simulink model "FL_simulink"  (R2023b)
settings: Solver=VariableStepAuto  StartTime=0.0  StopTime=30  RelTol=1e-3
values from neighbouring files (symbols this model uses):
  g = 9.81    [ASMC_with_sensor_noise_matlab.m]    (also in ASMC_without_sensor_noise_matlab.m; FL_matlab.m)
  k1 = K(1,1)    [ASMC_with_sensor_noise_matlab.m]    (also in ASMC_without_sensor_noise_matlab.m; FL_matlab.m = K(1))
  k2 = K(2,2)    [ASMC_with_sensor_noise_matlab.m]    (also in ASMC_without_sensor_noise_matlab.m; FL_matlab.m = K(2))
  k3 = K(3,3)    [ASMC_with_sensor_noise_matlab.m]    (also in ASMC_without_sensor_noise_matlab.m; FL_matlab.m = K(3))
  k4 = K(4,4)    [ASMC_with_sensor_noise_matlab.m]    (also in ASMC_without_sensor_noise_matlab.m; FL_matlab.m = K(4))
  k_psi1 = 30    [FL_matlab.m]
  k_psi2 = 50    [FL_matlab.m]
  l = 1    [ASMC_with_sensor_noise_matlab.m]    (also in ASMC_without_sensor_noise_matlab.m; FL_matlab.m)
  phi_0 = pi/6    (= 0.523598775598)    [ASMC_with_sensor_noise_matlab.m]    (also in ASMC_without_sensor_noise_matlab.m; FL_matlab.m)
  psi_0 = pi/6    (= 0.523598775598)    [ASMC_with_sensor_noise_matlab.m]    (also in ASMC_without_sensor_noise_matlab.m; FL_matlab.m)
  psi_d = 0    [ASMC_with_sensor_noise_matlab.m]    (also in ASMC_without_sensor_noise_matlab.m; FL_matlab.m)
  theta_0 = pi/6    (= 0.523598775598)    [ASMC_with_sensor_noise_matlab.m]    (also in ASMC_without_sensor_noise_matlab.m; FL_matlab.m)
  x_0 = 10    [ASMC_with_sensor_noise_matlab.m]    (also in ASMC_without_sensor_noise_matlab.m; FL_matlab.m)
  x_d1 = 20    [ASMC_with_sensor_noise_matlab.m]    (also in ASMC_without_sensor_noise_matlab.m; FL_matlab.m)
  x_d2 = 0    [ASMC_with_sensor_noise_matlab.m]    (also in ASMC_without_sensor_noise_matlab.m; FL_matlab.m)
  y_0 = 10    [ASMC_with_sensor_noise_matlab.m]    (also in ASMC_without_sensor_noise_matlab.m; FL_matlab.m)
  y_d1 = -10    [ASMC_with_sensor_noise_matlab.m]    (also in ASMC_without_sensor_noise_matlab.m; FL_matlab.m)
  y_d2 = 0    [ASMC_with_sensor_noise_matlab.m]    (also in ASMC_without_sensor_noise_matlab.m; FL_matlab.m)
  z_0 = 20    [ASMC_with_sensor_noise_matlab.m]    (also in ASMC_without_sensor_noise_matlab.m; FL_matlab.m)
  z_d1 = 10    [ASMC_with_sensor_noise_matlab.m]    (also in ASMC_without_sensor_noise_matlab.m; FL_matlab.m)
  z_d2 = 0    [ASMC_with_sensor_noise_matlab.m]    (also in ASMC_without_sensor_noise_matlab.m; FL_matlab.m)
settings Model: Creator=Kong Youngkyoung  LastModifiedBy=Kong Youngkyoung

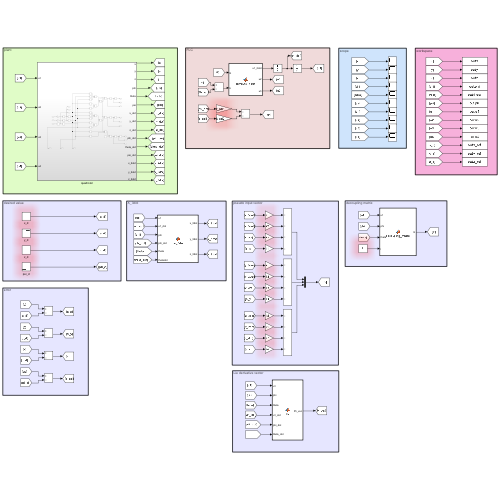
[thumbnail: Simulink's stored preview of the top-level diagram]
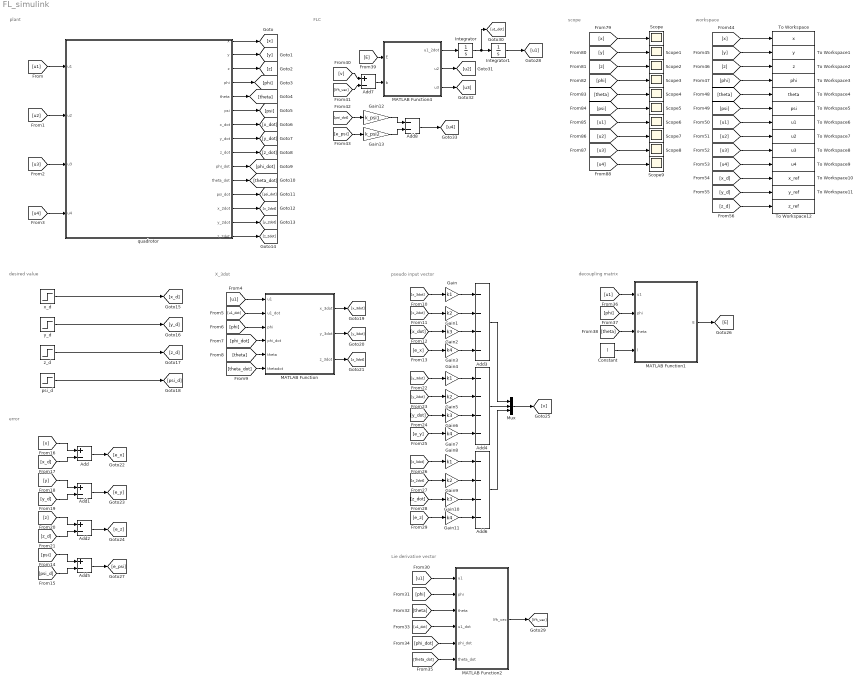
== system FL_simulink ==
  note: workspace
  note: decoupling matrix
  note: Lie derivative vector
  note: pseudo input vector
  note: X_3dot
  note: plant
  note: desired value
  note: error
  note: FLC
  note: scope
  Add{,1..2,5,7} (5 alike) : Sum  Inputs=+-
  Add3 : Sum  Inputs=----
  Add4 : Sum  Inputs=----
  Add6 : Sum  Inputs=----
  Add8 : Sum  Inputs=--
  Constant : Constant  Value=l
  Gain : Gain  Gain=k1
  Gain1 : Gain  Gain=k2
  Gain10 : Gain  Gain=k3
  Gain11 : Gain  Gain=k4
  Gain12 : Gain  Gain=k_psi1
  Gain13 : Gain  Gain=k_psi2
  Gain2 : Gain  Gain=k3
  Gain3 : Gain  Gain=k4
  Gain4 : Gain  Gain=k1
  Gain5 : Gain  Gain=k2
  Gain6 : Gain  Gain=k3
  Gain7 : Gain  Gain=k4
  Gain8 : Gain  Gain=k1
  Gain9 : Gain  Gain=k2
  Integrator : Integrator
  Integrator1 : Integrator  InitialCondition=0.0001
  MATLAB Function : MATLAB Function  TreatAsAtomicUnit=on
  MATLAB Function1 : MATLAB Function  TreatAsAtomicUnit=on
  MATLAB Function2 : MATLAB Function  TreatAsAtomicUnit=on
  MATLAB Function4 : MATLAB Function  TreatAsAtomicUnit=on
  Mux : Mux  Inputs=3
  Scope{,1..9} (10 alike) : Scope
  To Workspace : ToWorkspace  VariableName=x  SaveFormat=Timeseries  SampleTime=-1
  To Workspace1 : ToWorkspace  VariableName=y  SaveFormat=Timeseries  SampleTime=-1
  To Workspace10 : ToWorkspace  VariableName=x_ref  SaveFormat=Timeseries  SampleTime=-1
  To Workspace11 : ToWorkspace  VariableName=y_ref  SaveFormat=Timeseries  SampleTime=-1
  To Workspace12 : ToWorkspace  VariableName=z_ref  SaveFormat=Timeseries  SampleTime=-1
  To Workspace2 : ToWorkspace  VariableName=z  SaveFormat=Timeseries  SampleTime=-1
  To Workspace3 : ToWorkspace  VariableName=phi  SaveFormat=Timeseries  SampleTime=-1
  To Workspace4 : ToWorkspace  VariableName=theta  SaveFormat=Timeseries  SampleTime=-1
  To Workspace5 : ToWorkspace  VariableName=psi  SaveFormat=Timeseries  SampleTime=-1
  To Workspace6 : ToWorkspace  VariableName=u1  SaveFormat=Timeseries  SampleTime=-1
  To Workspace7 : ToWorkspace  VariableName=u2  SaveFormat=Timeseries  SampleTime=-1
  To Workspace8 : ToWorkspace  VariableName=u3  SaveFormat=Timeseries  SampleTime=-1
  To Workspace9 : ToWorkspace  VariableName=u4  SaveFormat=Timeseries  SampleTime=-1
  psi_d : Step  Time=15  Before=psi_d  After=psi_d  SampleTime=0
  quadrotor : Subsystem
  x_d : Step  Time=15  Before=x_d1  After=x_d2  SampleTime=0
  y_d : Step  Time=15  Before=y_d1  After=y_d2  SampleTime=0
  z_d : Step  Time=15  Before=z_d1  After=z_d2  SampleTime=0
  wires:
  quadrotor/14(y_2dot) -> [y_2dot]
  quadrotor/8(y_dot) -> [y_dot]
  quadrotor/5(theta) -> [theta]
  quadrotor/13(x_2dot) -> [x_2dot]
  quadrotor/10(phi_dot) -> [phi_dot]
  quadrotor/7(x_dot) -> [x_dot]
  quadrotor/3(z) -> [z]
  [u1] -> quadrotor/1(u1)
  quadrotor/11(theta_dot) -> [theta_dot]
  quadrotor/12(psi_dot) -> [psi_dot]
  quadrotor/9(z_dot) -> [z_dot]
  [u2] -> quadrotor/2(u2)
  quadrotor/15(z_2dot) -> [z_2dot]
  [u3] -> quadrotor/3(u3)
  quadrotor/6(psi) -> [psi]
  [u4] -> quadrotor/4(u4)
  quadrotor/2(y) -> [y]
  quadrotor/1(x) -> [x]
  quadrotor/4(phi) -> [phi]
  psi_d/1 -> [psi_d]
  x_d/1 -> [x_d]
  z_d/1 -> [z_d]
  y_d/1 -> [y_d]
  [theta] -> MATLAB Function/5(theta)
  [theta_dot] -> MATLAB Function/6(thetadot)
  [phi_dot] -> MATLAB Function/4(phi_dot)
  [phi] -> MATLAB Function/3(phi)
  [u1_dot] -> MATLAB Function/2(u1_dot)
  [u1] -> MATLAB Function/1(u1)
  MATLAB Function/1(x_3dot) -> [x_3dot]
  MATLAB Function/2(y_3dot) -> [y_3dot]
  MATLAB Function/3(z_3dot) -> [z_3dot]
  [z_d] -> Add2/2
  Add2/1 -> [e_z]
  Add/1 -> [e_x]
  Add1/1 -> [e_y]
  Add5/1 -> [e_psi]
  [psi_d] -> Add5/2
  [psi] -> Add5/1
  [y_d] -> Add1/2
  [z] -> Add2/1
  [x_d] -> Add/2
  [x] -> Add/1
  [y] -> Add1/1
  Gain/1 -> Add3/1
  Gain1/1 -> Add3/2
  Gain2/1 -> Add3/3
  Gain3/1 -> Add3/4
  [x_3dot] -> Gain/1
  [x_2dot] -> Gain1/1
  [x_dot] -> Gain2/1
  [e_x] -> Gain3/1
  Gain6/1 -> Add4/3
  Gain7/1 -> Add4/4
  [e_y] -> Gain7/1
  Gain4/1 -> Add4/1
  Gain5/1 -> Add4/2
  [y_2dot] -> Gain5/1
  Add4/1 -> Mux/2
  [y_dot] -> Gain6/1
  [y_3dot] -> Gain4/1
  Gain10/1 -> Add6/3
  Gain11/1 -> Add6/4
  [e_z] -> Gain11/1
  Gain8/1 -> Add6/1
  Gain9/1 -> Add6/2
  [z_2dot] -> Gain9/1
  Add6/1 -> Mux/3
  [z_dot] -> Gain10/1
  [z_3dot] -> Gain8/1
  [u1] -> MATLAB Function2/1(u1)
  [phi] -> MATLAB Function2/2(phi)
  [theta] -> MATLAB Function2/3(theta)
  [u1_dot] -> MATLAB Function2/4(u1_dot)
  [phi_dot] -> MATLAB Function2/5(phi_dot)
  [theta_dot] -> MATLAB Function2/6(theta_dot)
  MATLAB Function2/1(lfh_vec) -> [lfh_vec]
  Add3/1 -> Mux/1
  Mux/1 -> [v]
  Constant/1 -> MATLAB Function1/4(l)
  [theta] -> MATLAB Function1/3(theta)
  [phi] -> MATLAB Function1/2(phi)
  [u1] -> MATLAB Function1/1(u1)
  MATLAB Function1/1(E) -> [E]
  Add7/1 -> MATLAB Function4/2(b)
  [v] -> Add7/1
  [lfh_vec] -> Add7/2
  [E] -> MATLAB Function4/1(E)
  MATLAB Function4/1(u1_2dot) -> Integrator/1
  Integrator/1 -> [u1_dot], Integrator1/1
  Integrator1/1 -> [u1]
  MATLAB Function4/2(u2) -> [u2]
  MATLAB Function4/3(u3) -> [u3]
  [psi_dot] -> Gain12/1
  [e_psi] -> Gain13/1
  Gain12/1 -> Add8/1
  Gain13/1 -> Add8/2
  Add8/1 -> [u4]
  [z] -> Scope2/1
  [theta] -> Scope4/1
  [u3] -> Scope8/1
  [u1] -> Scope6/1
  [x] -> Scope/1
  [y] -> Scope1/1
  [phi] -> Scope3/1
  [u2] -> Scope7/1
  [u4] -> Scope9/1
  [psi] -> Scope5/1
  [psi] -> To Workspace5/1
  [z] -> To Workspace2/1
  [u2] -> To Workspace7/1
  [phi] -> To Workspace3/1
  [u1] -> To Workspace6/1
  [theta] -> To Workspace4/1
  [u4] -> To Workspace9/1
  [y] -> To Workspace1/1
  [u3] -> To Workspace8/1
  [x] -> To Workspace/1
  [x_d] -> To Workspace10/1
  [y_d] -> To Workspace11/1
  [z_d] -> To Workspace12/1

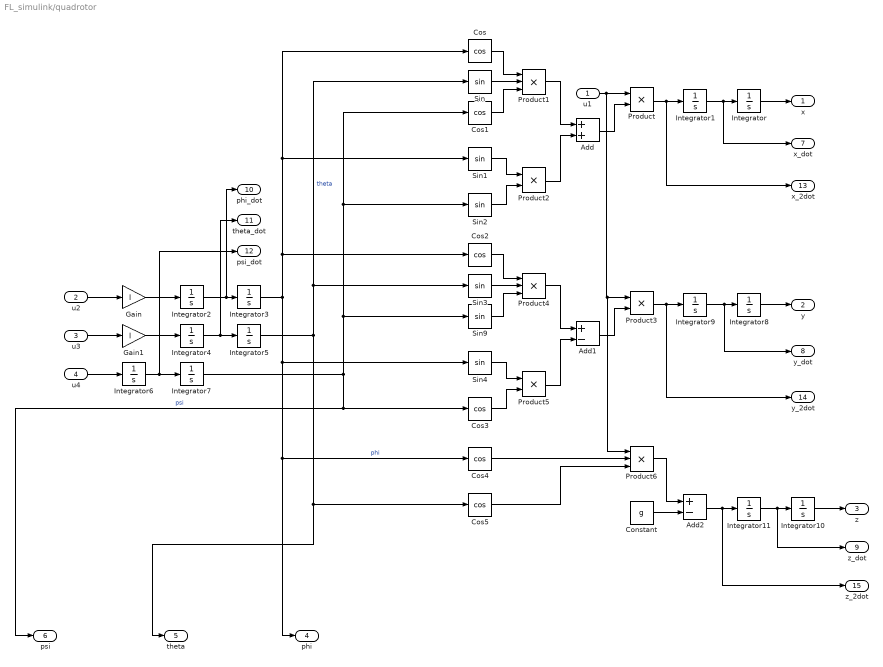
== system FL_simulink/quadrotor ==
  u1 : Inport
  u2 : Inport  Port=2
  u3 : Inport  Port=3
  u4 : Inport  Port=4
  Add : Sum
  Add1 : Sum  Inputs=+-
  Add2 : Sum  Inputs=+-
  Constant : Constant  Value=g
  Cos{,1..5} (6 alike) : Trigonometry  Operator=cos
  Gain : Gain  Gain=l
  Gain1 : Gain  Gain=l
  Integrator : Integrator  InitialCondition=x_0
  Integrator{1..2,4,6,9,11} (6 alike) : Integrator
  Integrator10 : Integrator  InitialCondition=z_0
  Integrator3 : Integrator  InitialCondition=phi_0
  Integrator5 : Integrator  InitialCondition=theta_0
  Integrator7 : Integrator  InitialCondition=psi_0
  Integrator8 : Integrator  InitialCondition=y_0
  Product{,2..3,5} (4 alike) : Product
  Product1 : Product  Inputs=3
  Product4 : Product  Inputs=3
  Product6 : Product  Inputs=3
  Sin{,1..4,9} (6 alike) : Trigonometry
  x : Outport
  y : Outport  Port=2
  z : Outport  Port=3
  phi : Outport  Port=4
  theta : Outport  Port=5
  psi : Outport  Port=6
  x_dot : Outport  Port=7
  y_dot : Outport  Port=8
  z_dot : Outport  Port=9
  phi_dot : Outport  Port=10
  theta_dot : Outport  Port=11
  psi_dot : Outport  Port=12
  x_2dot : Outport  Port=13
  y_2dot : Outport  Port=14
  z_2dot : Outport  Port=15
  wires:
  Integrator1/1 -> x_dot/1, Integrator/1
  Product/1 -> x_2dot/1, Integrator1/1
  u1/1 -> Product/1, Product6/1, Product3/1
  Add/1 -> Product/2
  Product1/1 -> Add/1
  Product2/1 -> Add/2
  Cos/1 -> Product1/1
  Sin/1 -> Product1/2
  Cos1/1 -> Product1/3
  Sin2/1 -> Product2/2
  Sin1/1 -> Product2/1
  u2/1 -> Gain/1
  u3/1 -> Gain1/1
  Gain/1 -> Integrator2/1
  Integrator2/1 -> phi_dot/1, Integrator3/1
  Integrator3/1 -> Cos4/1, phi/1, Sin4/1, Cos2/1, Cos/1, Sin1/1  "phi"
  Integrator5/1 -> theta/1, Cos5/1, Sin3/1, Sin/1  "theta"
  Gain1/1 -> Integrator4/1
  Integrator4/1 -> theta_dot/1, Integrator5/1
  Integrator7/1 -> psi/1, Cos3/1, Sin9/1, Sin2/1, Cos1/1  "psi"
  u4/1 -> Integrator6/1
  Integrator6/1 -> psi_dot/1, Integrator7/1
  Cos3/1 -> Product5/2
  Product5/1 -> Add1/2
  Product3/1 -> y_2dot/1, Integrator9/1
  Product4/1 -> Add1/1
  Cos2/1 -> Product4/1
  Sin3/1 -> Product4/2
  Sin9/1 -> Product4/3
  Integrator9/1 -> y_dot/1, Integrator8/1
  Sin4/1 -> Product5/1
  Add1/1 -> Product3/2
  Integrator11/1 -> z_dot/1, Integrator10/1
  Product6/1 -> Add2/1
  Constant/1 -> Add2/2
  Cos4/1 -> Product6/2
  Cos5/1 -> Product6/3
  Add2/1 -> z_2dot/1, Integrator11/1
  Integrator/1 -> x/1
  Integrator8/1 -> y/1
  Integrator10/1 -> z/1

== matlab function FL_simulink/MATLAB Function1 ==
  data: u1 input; E output; phi input; theta input; l input
function E = decoupling_matrix(u1,phi,theta,l)

a11=sin(theta);
a12=0;
a13=u1*cos(theta)*l;
a21=-sin(phi);
a22=-u1*cos(phi)*l;
a23=0;
a31=cos(theta)*cos(phi);
a32=-u1*cos(theta)*sin(phi)*l;
a33=-u1*sin(theta)*cos(phi)*l;

E = [a11 a12 a13; a21 a22 a23; a31 a32 a33];

== matlab function FL_simulink/MATLAB Function2 ==
  data: u1 input; lfh_vec output; phi input; theta input; u1_dot input; phi_dot input; theta_dot input
function lfh_vec = lfh(u1,phi,theta,u1_dot,phi_dot,theta_dot)

w1 = 2*u1_dot*theta_dot*cos(theta)-u1*theta_dot^2*sin(theta);
w2 = -2*u1_dot*phi_dot*cos(phi)+u1*phi_dot^2*sin(phi);
w3 = -2*u1_dot*theta_dot*sin(theta)*cos(phi)-2*u1_dot*phi_dot*cos(theta)*sin(phi)+2*u1*theta_dot*phi_dot*sin(theta)*sin(phi)-u1*(theta_dot^2+phi_dot^2)*cos(theta)*cos(phi);
lfh_vec = [w1; w2; w3];

== matlab function FL_simulink/MATLAB Function4 ==
  data: E input; u1_2dot output; b input; u2 output; u3 output
function [u1_2dot, u2, u3] = compute_input(E,b)

input_vec = E\b;

u1_2dot=input_vec(1);
u2=input_vec(2);
u3 = input_vec(3);

== matlab function FL_simulink/MATLAB Function ==
  data: u1 input; x_3dot output; u1_dot input; phi input; phi_dot input; theta input; thetadot input; y_3dot output; z_3dot output
function [x_3dot, y_3dot, z_3dot] = pos_3dot(u1, u1_dot, phi, phi_dot, theta, thetadot)

x_3dot = u1_dot*sin(theta)+u1*thetadot*cos(theta);
y_3dot = -u1_dot*sin(phi)-u1*phi_dot*cos(phi);
z_3dot = u1_dot*cos(theta)*cos(phi)-u1*thetadot*sin(theta)*cos(phi)-u1*phi_dot*cos(theta)*sin(phi);
